simulink model "mensajes"  (R2023b)
settings: Solver=VariableStepAuto  StartTime=0.0  StopTime=10.0  RelTol=1e-3
settings Model: Creator=anruk  LastModifiedBy=anruk

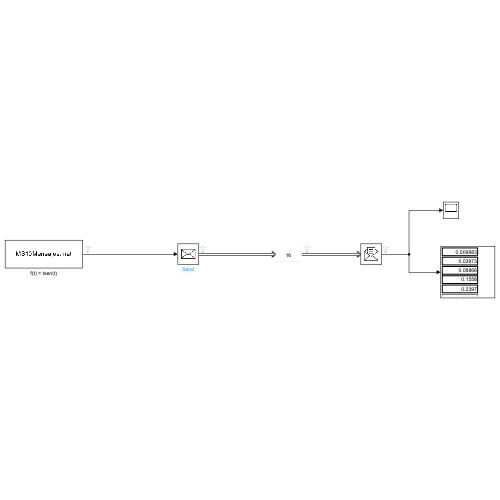
[thumbnail: Simulink's stored preview of the top-level diagram]
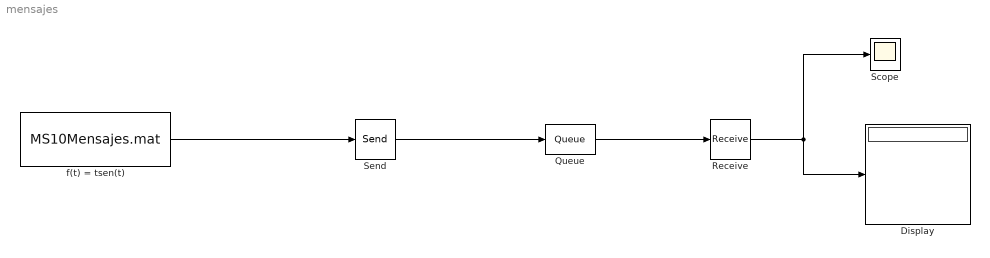
== system mensajes ==
  Display : Display
  Queue : Queue  InputPortMessageModes=m  OutputPortMessageModes=m  OverwriteOldest=on  Capacity=16  QueueType=LIFO
  Receive : Receive  InputPortMessageModes=m  UseInternalQueue=off  QueueOverwriting=on  QueueLength=1  QueueType=LIFO
  Scope : Scope
  Send : Send  OutputPortMessageModes=m
  f(t) = tsen(t) : FromFile  FileName=MS10Mensajes.mat  SampleTime=0
  wires:
  f(t) = tsen(t)/1 -> Send/1
  Send/1 -> Queue/1
  Queue/1 -> Receive/1
  Receive/1 -> Scope/1, Display/1
